simulink model "AdaptiveControlTrajectoryTracking"  (R2020b)
settings: Solver=VariableStepAuto  StartTime=0.0  StopTime=160  RelTol=1e-3
libraries: mobileRoboticsLib x4, simulink x4, dspinverses x4, dsppolyfun x4
settings Model: Creator=user  LastModifiedBy=user

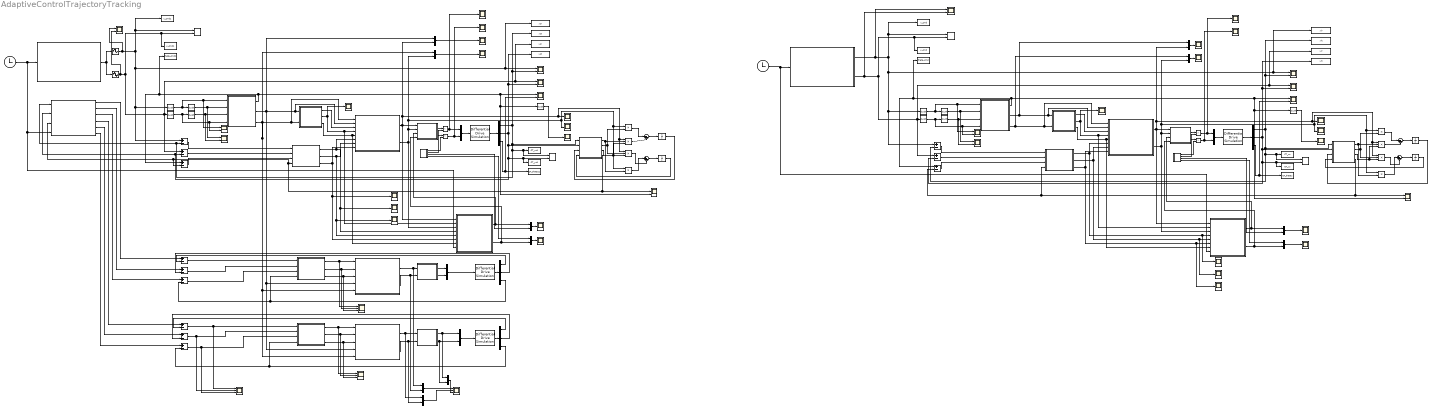
== system AdaptiveControlTrajectoryTracking ==
  Clock : Clock
  Clock1 : Clock
  Control law : MATLAB Function  TreatAsAtomicUnit=on
  Control law1 : MATLAB Function  TreatAsAtomicUnit=on
  Control law2 : MATLAB Function  TreatAsAtomicUnit=on
  Control law3 : MATLAB Function  TreatAsAtomicUnit=on
  Demux{1..4} (4 alike) : Demux  Outputs=3
  Derivative{1..10} (10 alike) : Derivative  CoefficientInTFapproximation=0
  Desired trajectory1 : MATLAB Function  TreatAsAtomicUnit=on
  Desired trajectory2 : MATLAB Function  TreatAsAtomicUnit=on
  Differential Drive Simulation1 : mobileRoboticsLib/Kinematic Models/Differential Drive/Differential Drive Simulation  wheelRadius=0.075  wheelBase=0.3  initX=0.05  initY=0.02  initAngle=pi-0.2  Ts=-1
      settings: SourceProductName=Mobile Robotics Simulation Toolbox
  Differential Drive Simulation2 : mobileRoboticsLib/Kinematic Models/Differential Drive/Differential Drive Simulation  wheelRadius=0.075  wheelBase=0.3  initX=0.2  initY=0.1  initAngle=pi  Ts=0.01
      settings: SourceProductName=Mobile Robotics Simulation Toolbox
  Differential Drive Simulation3 : mobileRoboticsLib/Kinematic Models/Differential Drive/Differential Drive Simulation  wheelRadius=0.075  wheelBase=0.3  initX=0.6  initY=-0.4  initAngle=pi  Ts=0.01
      settings: SourceProductName=Mobile Robotics Simulation Toolbox
  Differential Drive Simulation4 : mobileRoboticsLib/Kinematic Models/Differential Drive/Differential Drive Simulation  wheelRadius=0.075  wheelBase=0.3  initX=-0.15  initY=-0.13  initAngle=0  Ts=-1
      settings: SourceProductName=Mobile Robotics Simulation Toolbox
  Error1 : MATLAB Function  TreatAsAtomicUnit=on
  Error2 : MATLAB Function  TreatAsAtomicUnit=on
  Error3 : MATLAB Function  TreatAsAtomicUnit=on
  Error5 : MATLAB Function  TreatAsAtomicUnit=on
  Feedback gain1 : MATLAB Function  TreatAsAtomicUnit=on
  Feedback gain2 : MATLAB Function  TreatAsAtomicUnit=on
  Formation Control : MATLAB Function  TreatAsAtomicUnit=on
  Integrator : Integrator  InitialCondition=-100
  Integrator1 : Integrator  InitialCondition=1
  Integrator2 : Integrator  InitialCondition=800
  Integrator3 : Integrator  InitialCondition=200
  MATLAB Function1 : MATLAB Function  TreatAsAtomicUnit=on
  MATLAB Function2 : MATLAB Function  TreatAsAtomicUnit=on
  MATLAB Function3 : MATLAB Function  TreatAsAtomicUnit=on
  MATLAB Function4 : MATLAB Function  TreatAsAtomicUnit=on
  Mux{,1..11,14,17..18} (15 alike) : Mux  Inputs=2
  Observer : MATLAB Function  TreatAsAtomicUnit=on
  Observer slip{2..5} (4 alike) : Scope
  Observer theta : Scope  NumInputPorts=2
  Observer theta1 : Scope  NumInputPorts=2
  Observer theta3 : Scope
  Observer theta4 : Scope
  Observer1 : MATLAB Function  TreatAsAtomicUnit=on
  Product{,1..3,6..9} (8 alike) : Product
  Product{4..5,10..11} (4 alike) : Product  Inputs=3
  Scope{1,4,9..10} (4 alike) : Scope  NumInputPorts=2
  Scope{2..3,5..8,11..14} (10 alike) : Scope
  Subsystem1 : Subsystem
  Subsystem2 : Subsystem
  Subsystem3 : Subsystem
  Subsystem4 : Subsystem
  Sum : Sum  Inputs=|--
  Sum1 : Sum  Inputs=|+-
  Sum2 : Sum  Inputs=|--
  Sum3 : Sum  Inputs=|+-
  To Workspace : ToWorkspace  VariableName=xlr  SampleTime=.01
      settings: Save2DSignal=2-D array (concatenate along first dimension)
  To Workspace1 : ToWorkspace  VariableName=y_cmd  SampleTime=-1
      settings: Save2DSignal=2-D array (concatenate along first dimension)
  To Workspace10 : ToWorkspace  VariableName=y_cmd1  SampleTime=-1
      settings: Save2DSignal=2-D array (concatenate along first dimension)
  To Workspace11 : ToWorkspace  VariableName=theta_cmd1  SampleTime=-1
      settings: Save2DSignal=2-D array (concatenate along first dimension)
  To Workspace12 : ToWorkspace  VariableName=CT_thetas1  SampleTime=-1
      settings: Save2DSignal=2-D array (concatenate along first dimension)
  To Workspace13 : ToWorkspace  VariableName=xlt  SampleTime=.01
      settings: Save2DSignal=2-D array (concatenate along first dimension)
  To Workspace14 : ToWorkspace  VariableName=ylr  SampleTime=.01
      settings: Save2DSignal=2-D array (concatenate along first dimension)
  To Workspace15 : ToWorkspace  VariableName=ylt  SampleTime=.01
      settings: Save2DSignal=2-D array (concatenate along first dimension)
  To Workspace16 : ToWorkspace  VariableName=xcr  SampleTime=.01
      settings: Save2DSignal=2-D array (concatenate along first dimension)
  To Workspace17 : ToWorkspace  VariableName=xct  SampleTime=.01
      settings: Save2DSignal=2-D array (concatenate along first dimension)
  To Workspace18 : ToWorkspace  VariableName=ycr  SampleTime=.01
      settings: Save2DSignal=2-D array (concatenate along first dimension)
  To Workspace19 : ToWorkspace  VariableName=yct  SampleTime=.01
      settings: Save2DSignal=2-D array (concatenate along first dimension)
  To Workspace2 : ToWorkspace  VariableName=theta_cmd  SampleTime=-1
      settings: Save2DSignal=2-D array (concatenate along first dimension)
  To Workspace3 : ToWorkspace  VariableName=CT_xs1  SampleTime=-1
      settings: Save2DSignal=2-D array (concatenate along first dimension)
  To Workspace4 : ToWorkspace  VariableName=CT_ys1  SampleTime=-1
      settings: Save2DSignal=2-D array (concatenate along first dimension)
  To Workspace5 : ToWorkspace  VariableName=x_cmd1  SampleTime=-1
      settings: Save2DSignal=2-D array (concatenate along first dimension)
  To Workspace6 : ToWorkspace  VariableName=CT_thetas  SampleTime=-1
      settings: Save2DSignal=2-D array (concatenate along first dimension)
  To Workspace7 : ToWorkspace  VariableName=CT_xs  SampleTime=-1
      settings: Save2DSignal=2-D array (concatenate along first dimension)
  To Workspace8 : ToWorkspace  VariableName=CT_ys  SampleTime=-1
      settings: Save2DSignal=2-D array (concatenate along first dimension)
  To Workspace9 : ToWorkspace  VariableName=x_cmd  SampleTime=-1
      settings: Save2DSignal=2-D array (concatenate along first dimension)
  XY Graph desire1 : simulink/Sinks/XY Graph  xmin=-4  xmax=4  ymin=-4  ymax=4  st=-1
  XY Graph desire2 : simulink/Sinks/XY Graph  xmin=-1  xmax=10  ymin=-1  ymax=10  st=-1
  XY Graph tracking1 : simulink/Sinks/XY Graph  xmin=-4  xmax=4  ymin=-4  ymax=4  st=-1
  XY Graph tracking2 : simulink/Sinks/XY Graph  xmin=-1  xmax=10  ymin=-1  ymax=10  st=-1
  Xd1 : Sin  TimeSource=Use external signal  Amplitude=-1.6  SampleTime=0
  Yd1 : Sin  TimeSource=Use external signal  Amplitude=-1.6  Bias=1.6  Phase=pi/2  SampleTime=0
  angular velocity1 : Scope
  angular velocity2 : Scope
  dtheta1 : Scope
  dtheta2 : Scope
  e{1..4} (4 alike) : Scope
  error{1..4} (4 alike) : Scope  NumInputPorts=3
  left d1 : Scope  NumInputPorts=2
  left d2 : Scope  NumInputPorts=2
  theta1 : Scope  NumInputPorts=2
  theta2 : Scope  NumInputPorts=2
  theta_err{1..3,5} (4 alike) : Sum  Inputs=+-
  trajectory1 : Subsystem
  trajectory2 : Subsystem
  velocity1 : Scope
  velocity2 : Scope
  x1 : Scope  NumInputPorts=2
  x2 : Scope  NumInputPorts=2
  x_err{1..3,5} (4 alike) : Sum  Inputs=+-
  y1 : Scope  NumInputPorts=2
  y2 : Scope  NumInputPorts=2
  y_err{1..3,5} (4 alike) : Sum  Inputs=+-
  wires:
  Mux14/1 -> Observer slip2/1
  Mux/1 -> Observer slip3/1
  Subsystem2/1(ir) -> Product/2
  Feedback gain2/1(k1) -> Control law/3(k1)
  Mux1/1 -> Differential Drive Simulation1/1
  y_err2/1 -> Error2/2(y_err)
  Yd1/1 -> Scope10/2, To Workspace18/1, y2/1, Derivative5/1, y_err2/1, XY Graph desire1/2, To Workspace10/1
  Derivative5/1 -> Desired trajectory2/4(yd_d), left d1/2, Derivative8/1  "yd_d"
  Xd1/1 -> Scope10/1, To Workspace16/1, x2/1, Derivative4/1, x_err2/1, To Workspace5/1, XY Graph desire1/1
  Product/1 -> Mux1/2, Scope11/1
  Clock/1 -> Subsystem3/8(t), Formation Control/4(time), trajectory1/1(In1)
  Subsystem2/3(pl) -> Mux/2
  Subsystem3/1(Pl_hat) -> MATLAB Function1/3(Pl_hat), Mux/1
  theta_err2/1 -> Error2/3(theta_error)
  Desired trajectory2/1(td) -> To Workspace11/1, theta_err2/1, theta2/1, Observer theta/2, Derivative9/1
  Subsystem2/4(pr) -> Mux14/1
  Desired trajectory2/2(vd) -> Control law2/4(vd), Control law1/4(vd), Mux6/1, Feedback gain2/1(vd), Control law/2(vd)  "vr"
  Control law/1(v) -> MATLAB Function1/1(v), Product5/1, Product4/1, velocity1/1, Mux6/2, Subsystem3/1(v)  "v"
  Feedback gain2/2(k2) -> Scope14/1, Subsystem3/2(k2), Control law/4(k2)
  Product1/1 -> Mux1/1, Scope7/1
  MATLAB Function1/2(wr) -> Product/1  "wr"
  MATLAB Function1/1(wl) -> Product1/1  "wl"
  Differential Drive Simulation1/1 -> Demux1/1
  Subsystem2/2(il) -> Product1/2
  Derivative4/1 -> Derivative6/1, left d1/1, Desired trajectory2/1(xd_d)  "xd_d"
  Feedback gain2/3(k3) -> Control law/5(k3), Subsystem3/7(k3)
  Subsystem3/2(Pr_hat) -> MATLAB Function1/4(Pr_hat), Mux14/2
  trajectory1/1(Out1) -> Yd1/1, Xd1/1
  Derivative8/1 -> Scope9/2, Desired trajectory2/3(yd_dd)  "yd_dd"
  x_err2/1 -> Error2/1(x_err)
  Derivative6/1 -> Scope9/1, Desired trajectory2/2(xd_dd)  "xd_dd"
  Derivative9/1 -> dtheta1/1
  Control law/2(w) -> Mux7/2, Product3/1, Product2/1, angular velocity1/1, MATLAB Function1/2(w), Subsystem3/3(w)  "w"
  MATLAB Function2/1(wl) -> Mux2/1  "wl"
  MATLAB Function2/2(wr) -> Mux2/2  "wr"
  Control law1/1(v) -> MATLAB Function2/1(v), Mux4/1  "v"
  Control law1/2(w) -> MATLAB Function2/2(w), Mux4/2  "w"
  Differential Drive Simulation2/1 -> Demux2/1
  Control law2/2(w) -> Mux5/2, MATLAB Function3/2(w)  "w"
  Differential Drive Simulation3/1 -> Demux3/1
  Control law2/1(v) -> Mux5/1, MATLAB Function3/1(v)  "v"
  Error1/1(e1) -> error4/1, Control law1/1(ex)
  Error1/2(e2) -> error4/2, Control law1/2(ey)
  Error3/1(e1) -> error1/1, Control law2/1(ex)
  Error3/2(e2) -> error1/2, Control law2/2(ey)
  Error3/3(e3) -> error1/3, Control law2/3(et)
  x_err1/1 -> Error1/1(x_err)
  y_err1/1 -> Error1/2(y_err)
  theta_err1/1 -> Error1/3(theta_error)
  x_err3/1 -> error3/1, Error3/1(x_err)
  y_err3/1 -> error3/2, Error3/2(y_err)
  theta_err3/1 -> error3/3, Error3/3(theta_error)
  Demux3/3 -> Error3/4(theta), theta_err3/2
  Demux2/1 -> x_err1/2
  Demux2/2 -> y_err1/2
  Demux2/3 -> Error1/4(theta), theta_err1/2
  Formation Control/1(fx1) -> x_err1/1
  Formation Control/2(fy1) -> y_err1/1
  Formation Control/3(ft1) -> theta_err1/1
  Formation Control/4(fx2) -> x_err3/1
  Formation Control/5(fy2) -> y_err3/1
  Formation Control/6(fz2) -> theta_err3/1
  Mux4/1 -> error2/1
  Mux5/1 -> error2/2
  Demux1/1 -> XY Graph tracking1/1, To Workspace3/1, x_err2/2, Formation Control/1(Lx), Observer/1(z1), To Workspace17/1, x2/2
  Demux1/3 -> theta2/2, To Workspace12/1
  Demux1/2 -> To Workspace4/1, XY Graph tracking1/2, y_err2/2, Formation Control/2(Ly), Observer/2(z2), To Workspace19/1, y2/2
  Mux3/1 -> Differential Drive Simulation3/1
  Mux2/1 -> Differential Drive Simulation2/1
  MATLAB Function3/1(wl) -> Mux3/1, Mux8/1
  MATLAB Function3/2(wr) -> Mux3/2, Mux8/2
  Mux8/1 -> error2/3
  Demux3/2 -> y_err3/2
  Demux3/1 -> x_err3/2
  Error1/3(e3) -> error4/3, Control law1/3(et)
  Desired trajectory2/3(wd) -> Control law/1(wd), Feedback gain2/2(wd), Control law2/5(wd), Control law1/5(wd), Mux7/1  "wr"
  Observer/1(z3_hat) -> Product2/2, Product4/2
  Observer/3(L) -> Product5/3, Product4/3
  Observer/2(z4_hat) -> Product5/2, Product3/2
  Product3/1 -> Sum/1
  Product4/1 -> Sum/2
  Product2/1 -> Sum1/1
  Product5/1 -> Sum1/2
  Sum/1 -> Integrator/1
  Sum1/1 -> Integrator1/1
  Integrator/1 -> Observer/3(alpha)
  Integrator1/1 -> Observer/4(beta)
  Observer/4(theta) -> theta_err2/2, Formation Control/3(Lt), Error2/4(theta), Observer theta/1
  Demux4/3 -> theta1/2, To Workspace6/1
  trajectory2/2(Out2) -> y1/1, To Workspace14/1, Derivative2/1, y_err5/1, XY Graph desire2/2, To Workspace1/1, Scope1/2
  Demux4/1 -> XY Graph tracking2/1, To Workspace7/1, x_err5/2, Observer1/1(z1), x1/2, To Workspace13/1
  Demux4/2 -> To Workspace8/1, XY Graph tracking2/2, y_err5/2, Observer1/2(z2), y1/2, To Workspace15/1
  Mux10/1 -> Differential Drive Simulation4/1
  Subsystem4/2(Pr_hat) -> MATLAB Function4/4(Pr_hat), Mux11/2
  MATLAB Function4/1(wl) -> Product7/1  "wl"
  MATLAB Function4/2(wr) -> Product6/1  "wr"
  Derivative10/1 -> dtheta2/1
  Feedback gain1/2(k2) -> Scope2/1, Subsystem4/2(k2), Control law3/4(k2)
  trajectory2/1(Out1) -> Scope1/1, To Workspace9/1, XY Graph desire2/1, x1/1, To Workspace/1, Derivative1/1, x_err5/1
  Control law3/2(w) -> Mux18/2, Product9/1, Product8/1, angular velocity2/1, MATLAB Function4/2(w), Subsystem4/3(w)  "w"
  Desired trajectory1/1(td) -> To Workspace2/1, theta_err5/1, theta1/1, Observer theta1/2, Derivative10/1
  Error5/1(e1) -> e1/1, Subsystem4/4(e1), Control law3/6(e1)  "e1"
  x_err5/1 -> Error5/1(x_err)
  Subsystem4/1(Pl_hat) -> Mux9/1, MATLAB Function4/3(Pl_hat)
  Derivative7/1 -> Scope4/2, Desired trajectory1/3(yd_dd)  "yd_dd"
  Derivative3/1 -> Scope4/1, Desired trajectory1/2(xd_dd)  "xd_dd"
  Control law3/1(v) -> MATLAB Function4/1(v), Product11/1, Product10/1, velocity2/1, Mux17/2, Subsystem4/1(v)  "v"
  Differential Drive Simulation4/1 -> Demux4/1
  Subsystem1/4(pr) -> Mux11/1
  Feedback gain1/3(k3) -> Control law3/5(k3), Subsystem4/7(k3)
  Desired trajectory1/2(vd) -> Mux17/1, Feedback gain1/1(vd), Control law3/2(vd)  "vr"
  Derivative1/1 -> Derivative3/1, left d2/1, Desired trajectory1/1(xd_d)  "xd_d"
  Feedback gain1/1(k1) -> Control law3/3(k1)
  Error5/3(e3) -> Control law3/8(e3), Observer theta3/1, Subsystem4/6(e3)  "e3"
  Subsystem1/3(pl) -> Mux9/2
  Subsystem1/1(ir) -> Product6/2
  theta_err5/1 -> Error5/3(theta_error)
  Mux18/1 -> Scope5/1
  Observer1/4(theta) -> Error5/4(theta), theta_err5/2, Observer theta1/1
  Mux17/1 -> Scope3/1
  Integrator2/1 -> Observer1/3(alpha)
  Mux9/1 -> Observer slip5/1
  Derivative2/1 -> Desired trajectory1/4(yd_d), left d2/2, Derivative7/1  "yd_d"
  Subsystem1/2(il) -> Product7/2
  Clock1/1 -> Subsystem4/8(t), trajectory2/1(In1)
  Sum2/1 -> Integrator2/1
  Observer1/1(z3_hat) -> Product8/2, Product10/2
  Error5/2(e2) -> e2/1, Subsystem4/5(e2), Control law3/7(e2)  "e2"
  Sum3/1 -> Integrator3/1
  Mux11/1 -> Observer slip4/1
  Integrator3/1 -> Observer1/4(beta)
  Observer1/3(L) -> Product11/3, Product10/3
  Observer1/2(z4_hat) -> Product11/2, Product9/2
  Product8/1 -> Sum3/1
  Product11/1 -> Sum3/2
  y_err5/1 -> Error5/2(y_err)
  Product10/1 -> Sum2/2
  Product9/1 -> Sum2/1
  Desired trajectory1/3(wd) -> Control law3/1(wd), Feedback gain1/2(wd), Mux18/1  "wr"
  Error2/3(e3) -> Control law/8(e3), Subsystem3/6(e3), e3/1  "e3"
  Error2/1(e1) -> Subsystem3/4(e1), e4/1, Control law/6(e1)  "e1"
  Error2/2(e2) -> Control law/7(e2), Observer theta4/1, Subsystem3/5(e2)  "e2"
  Mux6/1 -> Scope6/1
  Mux7/1 -> Scope8/1
  Product6/1 -> Scope12/1, Mux10/2
  Product7/1 -> Scope13/1, Mux10/1

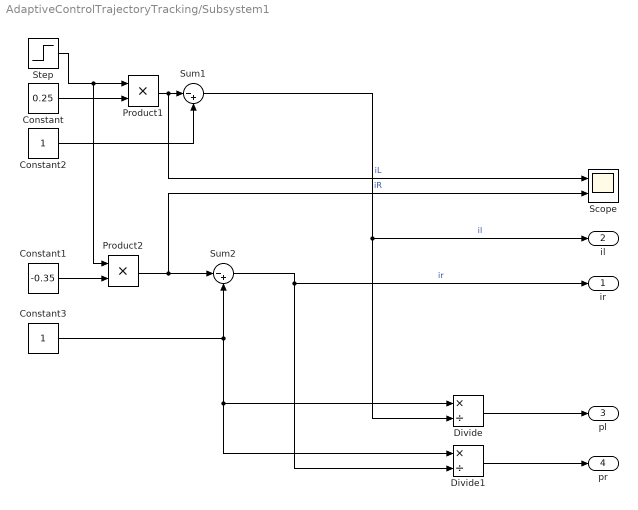
== system AdaptiveControlTrajectoryTracking/Subsystem1 ==
  Constant : Constant  Value=0.25
  Constant1 : Constant  Value=-0.35
  Constant2 : Constant
  Constant3 : Constant
  Divide : Product  Inputs=*/
  Divide1 : Product  Inputs=*/
  Product1 : Product
  Product2 : Product
  Scope : Scope  NumInputPorts=2
  Step : Step  Time=0  SampleTime=0
  Sum1 : Sum  Inputs=|-+
  Sum2 : Sum  Inputs=|-+
  ir : Outport
  il : Outport  Port=2
  pl : Outport  Port=3
  pr : Outport  Port=4
  wires:
  Sum1/1 -> Divide/2, il/1  "il"
  Step/1 -> Product2/1, Product1/1
  Constant3/1 -> Divide/1, Divide1/1, Sum2/2
  Product1/1 -> Scope/1, Sum1/1  "iL"
  Constant2/1 -> Sum1/2
  Sum2/1 -> ir/1, Divide1/2  "ir"
  Constant1/1 -> Product2/2
  Constant/1 -> Product1/2
  Product2/1 -> Scope/2, Sum2/1  "iR"
  Divide/1 -> pl/1
  Divide1/1 -> pr/1

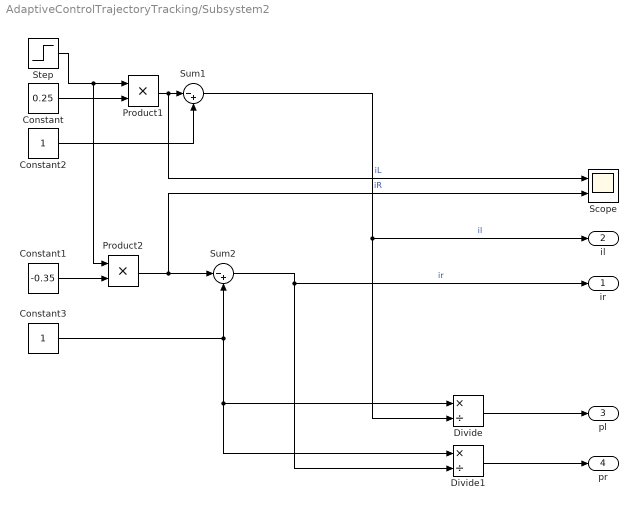
== system AdaptiveControlTrajectoryTracking/Subsystem2 ==
  Constant : Constant  Value=0.25
  Constant1 : Constant  Value=-0.35
  Constant2 : Constant
  Constant3 : Constant
  Divide : Product  Inputs=*/
  Divide1 : Product  Inputs=*/
  Product1 : Product
  Product2 : Product
  Scope : Scope  NumInputPorts=2
  Step : Step  Time=0  SampleTime=0
  Sum1 : Sum  Inputs=|-+
  Sum2 : Sum  Inputs=|-+
  ir : Outport
  il : Outport  Port=2
  pl : Outport  Port=3
  pr : Outport  Port=4
  wires:
  Sum1/1 -> Divide/2, il/1  "il"
  Step/1 -> Product2/1, Product1/1
  Constant3/1 -> Divide/1, Divide1/1, Sum2/2
  Product1/1 -> Scope/1, Sum1/1  "iL"
  Constant2/1 -> Sum1/2
  Sum2/1 -> ir/1, Divide1/2  "ir"
  Constant1/1 -> Product2/2
  Constant/1 -> Product1/2
  Product2/1 -> Scope/2, Sum2/1  "iR"
  Divide/1 -> pl/1
  Divide1/1 -> pr/1

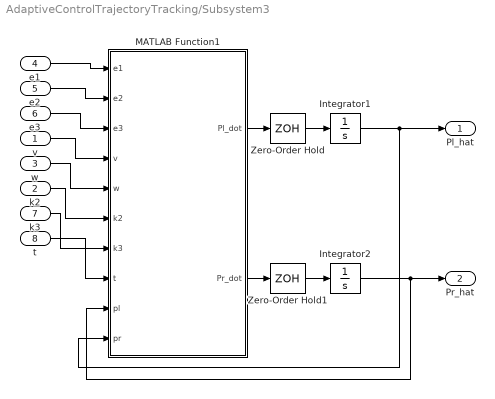
== system AdaptiveControlTrajectoryTracking/Subsystem3 ==
  v : Inport
  k2 : Inport  Port=2
  w : Inport  Port=3
  e1 : Inport  Port=4
  e2 : Inport  Port=5
  e3 : Inport  Port=6
  k3 : Inport  Port=7
  t : Inport  Port=8
  Integrator1 : Integrator  InitialCondition=1/0.85
  Integrator2 : Integrator  InitialCondition=1/1.2
  MATLAB Function1 : MATLAB Function  TreatAsAtomicUnit=on
  Zero-Order Hold : ZeroOrderHold  SampleTime=0.01
  Zero-Order Hold1 : ZeroOrderHold  SampleTime=0.01
  Pl_hat : Outport
  Pr_hat : Outport  Port=2
  wires:
  e2/1 -> MATLAB Function1/2(e2)
  Integrator1/1 -> Pl_hat/1, MATLAB Function1/10(pr)
  MATLAB Function1/2(Pr_dot) -> Zero-Order Hold1/1
  e3/1 -> MATLAB Function1/3(e3)
  w/1 -> MATLAB Function1/5(w)
  MATLAB Function1/1(Pl_dot) -> Zero-Order Hold/1
  k2/1 -> MATLAB Function1/6(k2)
  v/1 -> MATLAB Function1/4(v)
  e1/1 -> MATLAB Function1/1(e1)
  k3/1 -> MATLAB Function1/7(k3)
  Integrator2/1 -> Pr_hat/1, MATLAB Function1/9(pl)
  t/1 -> MATLAB Function1/8(t)
  Zero-Order Hold/1 -> Integrator1/1
  Zero-Order Hold1/1 -> Integrator2/1

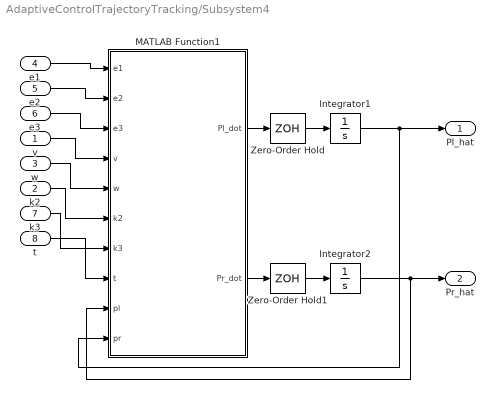
== system AdaptiveControlTrajectoryTracking/Subsystem4 ==
  v : Inport
  k2 : Inport  Port=2
  w : Inport  Port=3
  e1 : Inport  Port=4
  e2 : Inport  Port=5
  e3 : Inport  Port=6
  k3 : Inport  Port=7
  t : Inport  Port=8
  Integrator1 : Integrator  InitialCondition=1/0.85
  Integrator2 : Integrator  InitialCondition=1/1.2
  MATLAB Function1 : MATLAB Function  TreatAsAtomicUnit=on
  Zero-Order Hold : ZeroOrderHold  SampleTime=0.01
  Zero-Order Hold1 : ZeroOrderHold  SampleTime=0.01
  Pl_hat : Outport
  Pr_hat : Outport  Port=2
  wires:
  e2/1 -> MATLAB Function1/2(e2)
  Integrator1/1 -> Pl_hat/1, MATLAB Function1/10(pr)
  MATLAB Function1/2(Pr_dot) -> Zero-Order Hold1/1
  e3/1 -> MATLAB Function1/3(e3)
  w/1 -> MATLAB Function1/5(w)
  MATLAB Function1/1(Pl_dot) -> Zero-Order Hold/1
  k2/1 -> MATLAB Function1/6(k2)
  v/1 -> MATLAB Function1/4(v)
  e1/1 -> MATLAB Function1/1(e1)
  k3/1 -> MATLAB Function1/7(k3)
  Integrator2/1 -> Pr_hat/1, MATLAB Function1/9(pl)
  t/1 -> MATLAB Function1/8(t)
  Zero-Order Hold/1 -> Integrator1/1
  Zero-Order Hold1/1 -> Integrator2/1

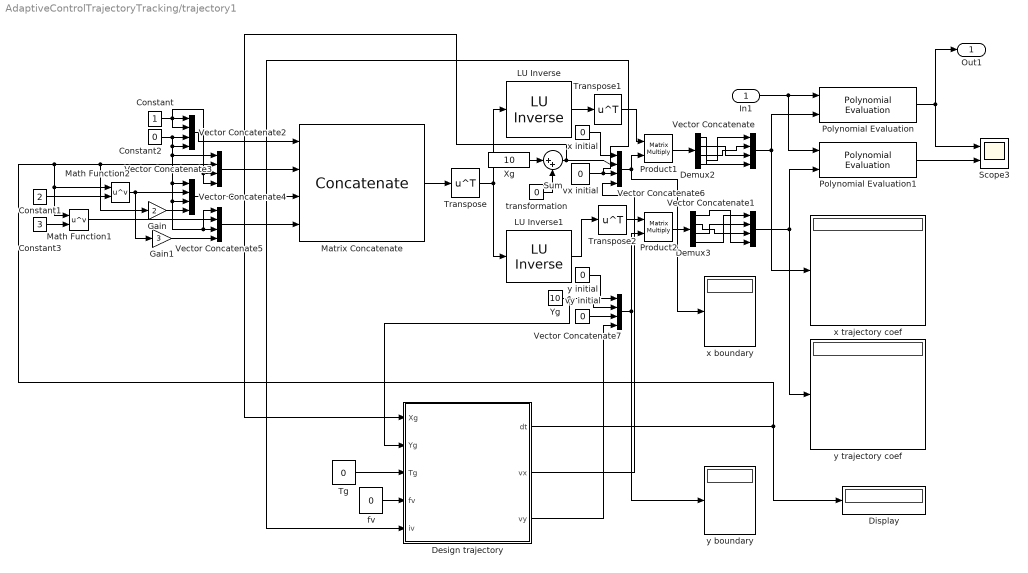
== system AdaptiveControlTrajectoryTracking/trajectory1 ==
  In1 : Inport
  " LU Inverse" : dspinverses/ LU Inverse
  " LU Inverse1" : dspinverses/ LU Inverse
  Constant : Constant
  Constant1 : Constant  Value=2
  Constant2 : Constant  Value=0
  Constant3 : Constant  Value=3
  Demux2 : Demux
  Demux3 : Demux
  Design trajectory : MATLAB Function  TreatAsAtomicUnit=on
  Display : Display
  Gain : Gain  Gain=2
  Gain1 : Gain  Gain=3
  Math Function1 : Math  Operator=pow  SaturateOnIntegerOverflow=on
  Math Function2 : Math  Operator=pow  SaturateOnIntegerOverflow=on
  Matrix Concatenate : Concatenate  NumInputs=4  Mode=Multidimensional array  ConcatenateDimension=2
  Polynomial Evaluation : dsppolyfun/Polynomial Evaluation  useConstCoeffs=off  constCoeffs=[5 4 3 2]
      settings: SourceProductBaseCode=DS
  Polynomial Evaluation1 : dsppolyfun/Polynomial Evaluation  useConstCoeffs=off  constCoeffs=[5 4 3 2]
      settings: SourceProductBaseCode=DS
  Product1 : Product  Multiplication=Matrix(*)
  Product2 : Product  Multiplication=Matrix(*)
  Scope3 : Scope  NumInputPorts=2
  Sum : Sum  Inputs=|++
  Tg : Constant  Value=0
  Transpose : Math  Operator=transpose  SaturateOnIntegerOverflow=on
  Transpose1 : Math  Operator=transpose  SaturateOnIntegerOverflow=on
  Transpose2 : Math  Operator=transpose  SaturateOnIntegerOverflow=on
  Vector Concatenate{,1..7} (8 alike) : Concatenate  NumInputs=4
  "Xg " : Constant  Value=10
  Yg : Constant  Value=10
  fv : Constant  Value=0
  transformation : Constant  Value=0
  "vx initial " : Constant  Value=0
  "vy initial " : Constant  Value=0
  "x boundary " : Display
  "x initial " : Constant  Value=0
  x trajectory coef : Display
  "y boundary " : Display
  "y initial " : Constant  Value=0
  y trajectory coef : Display
  Out1 : Outport
  wires:
  Polynomial Evaluation1/1 -> Scope3/2
  Product2/1 -> Demux3/1
  Yg/1 -> Design trajectory/2(Yg), Vector Concatenate7/2
  Math Function2/1 -> Gain1/1, Vector Concatenate4/2
  "vy initial "/1 -> Vector Concatenate7/3
  Tg/1 -> Design trajectory/3(Tg)
  Demux2/2 -> Vector Concatenate/3
  Constant/1 -> Vector Concatenate2/1, Vector Concatenate3/4, Vector Concatenate3/3, Vector Concatenate2/2
  fv/1 -> Design trajectory/4(fv)
  Vector Concatenate3/1 -> Matrix Concatenate/2
  Vector Concatenate5/1 -> Matrix Concatenate/4
  Vector Concatenate6/1 -> "x boundary "/1, Product1/2
  Vector Concatenate7/1 -> Product2/2, "y boundary "/1
  transformation/1 -> Sum/2
  Constant2/1 -> Vector Concatenate5/3, Vector Concatenate5/1, Vector Concatenate4/3, Vector Concatenate4/1, Vector Concatenate3/1, Vector Concatenate2/4, Vector Concatenate2/3
  Design trajectory/3(vy) -> Vector Concatenate7/4
  Transpose1/1 -> Product1/1
  "x initial "/1 -> Vector Concatenate6/1
  Demux3/4 -> Vector Concatenate1/1
  "Xg "/1 -> Sum/1
  " LU Inverse"/1 -> Transpose1/1
  " LU Inverse1"/1 -> Transpose2/1
  Product1/1 -> Demux2/1
  Vector Concatenate2/1 -> Matrix Concatenate/1
  "y initial "/1 -> Vector Concatenate7/1
  Demux2/3 -> Vector Concatenate/2
  Constant1/1 -> Math Function2/2
  Transpose2/1 -> Product2/1
  Matrix Concatenate/1 -> Transpose/1
  Vector Concatenate4/1 -> Matrix Concatenate/3
  Design trajectory/2(vx) -> Vector Concatenate6/4
  "vx initial "/1 -> Design trajectory/5(iv), Vector Concatenate6/3
  Polynomial Evaluation/1 -> Out1/1, Scope3/1
  Design trajectory/1(dt) -> Display/1, Math Function1/1, Math Function2/1, Vector Concatenate3/2, Gain/1
  Sum/1 -> Vector Concatenate6/2, Design trajectory/1(Xg)
  Transpose/1 -> " LU Inverse1"/1, " LU Inverse"/1
  In1/1 -> Polynomial Evaluation1/1, Polynomial Evaluation/1
  Constant3/1 -> Math Function1/2
  Math Function1/1 -> Vector Concatenate5/2
  Vector Concatenate1/1 -> y trajectory coef/1, Polynomial Evaluation1/2
  Gain/1 -> Vector Concatenate4/4
  Gain1/1 -> Vector Concatenate5/4
  Demux3/2 -> Vector Concatenate1/3
  Demux3/1 -> Vector Concatenate1/4
  Demux2/1 -> Vector Concatenate/4
  Demux3/3 -> Vector Concatenate1/2
  Vector Concatenate/1 -> x trajectory coef/1, Polynomial Evaluation/2
  Demux2/4 -> Vector Concatenate/1

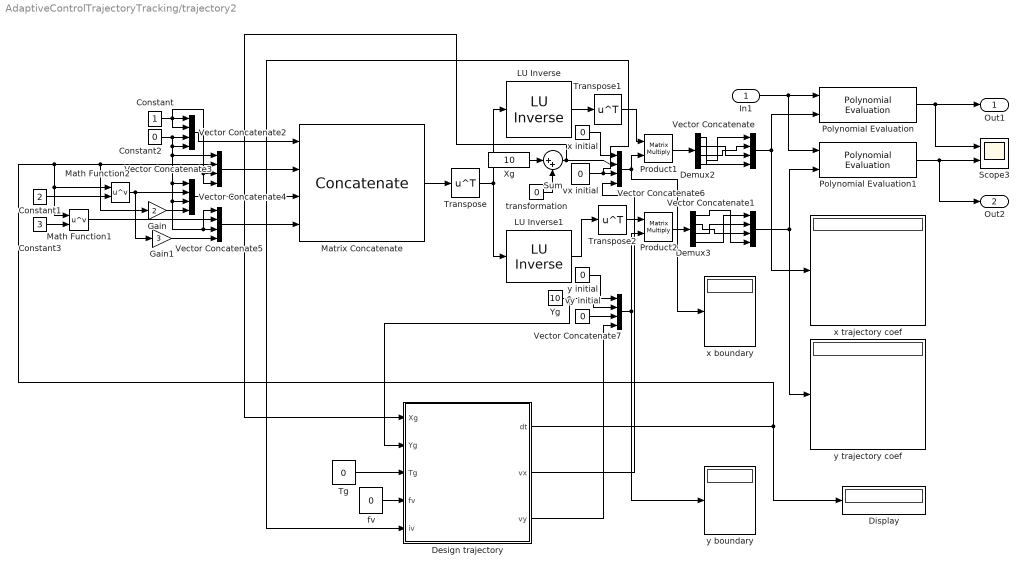
== system AdaptiveControlTrajectoryTracking/trajectory2 ==
  In1 : Inport
  " LU Inverse" : dspinverses/ LU Inverse
  " LU Inverse1" : dspinverses/ LU Inverse
  Constant : Constant
  Constant1 : Constant  Value=2
  Constant2 : Constant  Value=0
  Constant3 : Constant  Value=3
  Demux2 : Demux
  Demux3 : Demux
  Design trajectory : MATLAB Function  TreatAsAtomicUnit=on
  Display : Display
  Gain : Gain  Gain=2
  Gain1 : Gain  Gain=3
  Math Function1 : Math  Operator=pow  SaturateOnIntegerOverflow=on
  Math Function2 : Math  Operator=pow  SaturateOnIntegerOverflow=on
  Matrix Concatenate : Concatenate  NumInputs=4  Mode=Multidimensional array  ConcatenateDimension=2
  Polynomial Evaluation : dsppolyfun/Polynomial Evaluation  useConstCoeffs=off  constCoeffs=[5 4 3 2]
      settings: SourceProductBaseCode=DS
  Polynomial Evaluation1 : dsppolyfun/Polynomial Evaluation  useConstCoeffs=off  constCoeffs=[5 4 3 2]
      settings: SourceProductBaseCode=DS
  Product1 : Product  Multiplication=Matrix(*)
  Product2 : Product  Multiplication=Matrix(*)
  Scope3 : Scope  NumInputPorts=2
  Sum : Sum  Inputs=|++
  Tg : Constant  Value=0
  Transpose : Math  Operator=transpose  SaturateOnIntegerOverflow=on
  Transpose1 : Math  Operator=transpose  SaturateOnIntegerOverflow=on
  Transpose2 : Math  Operator=transpose  SaturateOnIntegerOverflow=on
  Vector Concatenate{,1..7} (8 alike) : Concatenate  NumInputs=4
  "Xg " : Constant  Value=10
  Yg : Constant  Value=10
  fv : Constant  Value=0
  transformation : Constant  Value=0
  "vx initial " : Constant  Value=0
  "vy initial " : Constant  Value=0
  "x boundary " : Display
  "x initial " : Constant  Value=0
  x trajectory coef : Display
  "y boundary " : Display
  "y initial " : Constant  Value=0
  y trajectory coef : Display
  Out1 : Outport
  Out2 : Outport  Port=2
  wires:
  Polynomial Evaluation1/1 -> Scope3/2, Out2/1
  Product2/1 -> Demux3/1
  Yg/1 -> Design trajectory/2(Yg), Vector Concatenate7/2
  Math Function2/1 -> Gain1/1, Vector Concatenate4/2
  "vy initial "/1 -> Vector Concatenate7/3
  Tg/1 -> Design trajectory/3(Tg)
  Demux2/2 -> Vector Concatenate/3
  Constant/1 -> Vector Concatenate2/1, Vector Concatenate3/4, Vector Concatenate3/3, Vector Concatenate2/2
  fv/1 -> Design trajectory/4(fv)
  Vector Concatenate3/1 -> Matrix Concatenate/2
  Vector Concatenate5/1 -> Matrix Concatenate/4
  Vector Concatenate6/1 -> "x boundary "/1, Product1/2
  Vector Concatenate7/1 -> Product2/2, "y boundary "/1
  transformation/1 -> Sum/2
  Constant2/1 -> Vector Concatenate5/3, Vector Concatenate5/1, Vector Concatenate4/3, Vector Concatenate4/1, Vector Concatenate3/1, Vector Concatenate2/4, Vector Concatenate2/3
  Design trajectory/3(vy) -> Vector Concatenate7/4
  Transpose1/1 -> Product1/1
  "x initial "/1 -> Vector Concatenate6/1
  Demux3/4 -> Vector Concatenate1/1
  "Xg "/1 -> Sum/1
  " LU Inverse"/1 -> Transpose1/1
  " LU Inverse1"/1 -> Transpose2/1
  Product1/1 -> Demux2/1
  Vector Concatenate2/1 -> Matrix Concatenate/1
  "y initial "/1 -> Vector Concatenate7/1
  Demux2/3 -> Vector Concatenate/2
  Constant1/1 -> Math Function2/2
  Transpose2/1 -> Product2/1
  Matrix Concatenate/1 -> Transpose/1
  Vector Concatenate4/1 -> Matrix Concatenate/3
  Design trajectory/2(vx) -> Vector Concatenate6/4
  "vx initial "/1 -> Design trajectory/5(iv), Vector Concatenate6/3
  Polynomial Evaluation/1 -> Out1/1, Scope3/1
  Design trajectory/1(dt) -> Display/1, Math Function1/1, Math Function2/1, Vector Concatenate3/2, Gain/1
  Sum/1 -> Vector Concatenate6/2, Design trajectory/1(Xg)
  Transpose/1 -> " LU Inverse1"/1, " LU Inverse"/1
  In1/1 -> Polynomial Evaluation1/1, Polynomial Evaluation/1
  Constant3/1 -> Math Function1/2
  Math Function1/1 -> Vector Concatenate5/2
  Vector Concatenate1/1 -> y trajectory coef/1, Polynomial Evaluation1/2
  Gain/1 -> Vector Concatenate4/4
  Gain1/1 -> Vector Concatenate5/4
  Demux3/2 -> Vector Concatenate1/3
  Demux3/1 -> Vector Concatenate1/4
  Demux2/1 -> Vector Concatenate/4
  Demux3/3 -> Vector Concatenate1/2
  Vector Concatenate/1 -> x trajectory coef/1, Polynomial Evaluation/2
  Demux2/4 -> Vector Concatenate/1

== matlab function AdaptiveControlTrajectoryTracking/Error3 ==
  data: x_err input; e1 output; y_err input; theta_error input; theta input; e2 output; e3 output
function [e1,e2,e3] = error(x_err,y_err,theta_error,theta)
    e=[cos(theta) sin(theta) 0;-sin(theta) cos(theta) 0;0 0 1]*[x_err;y_err;theta_error];
    e1=e(1);
    e2=e(2);
    e3=e(3);
end

== matlab function AdaptiveControlTrajectoryTracking/Error2 ==
  data: x_err input; e1 output; y_err input; theta_error input; theta input; e2 output; e3 output
function [e1,e2,e3] = error(x_err,y_err,theta_error,theta)
    e=[cos(theta) sin(theta) 0;-sin(theta) cos(theta) 0;0 0 1]*[x_err;y_err;theta_error];
    e1=e(1);
    e2=e(2);
    e3=e(3);
end

== matlab function AdaptiveControlTrajectoryTracking/Feedback gain2 ==
  data: k1 output; k2 output; k3 output; vd input; wd input
function [k1,k2,k3] = K(vd,wd)
    epsilon=1;
    kb=14;
    
    k1=2*epsilon*sqrt(wd^2+kb*vd^2);
    k3=k1;
    k2=kb*abs(vd);

end

== matlab function AdaptiveControlTrajectoryTracking/Control law ==
  data: wd input; vd input; v output; k1 input; k2 input; k3 input; e1 input; e2 input; e3 input; w output
function [v,w] = fcn(wd,vd,k1,k2,k3,e1,e2,e3)
    v=zeros(1);
    w=zeros(1);
    vmax=0.15;
    wmax=0.45;
    
    
%    vc=vd*cos(e3)+k1*e1;
%    wc=wd+k2*sign(vd)*e2+k3*e3;
    
    %% gain 
    
    k11 = 2;
    k22 = 10;
    k33 = 2;
    
    %%
    wc = wd + vd / 2 * (k22 * (e2 + k33 * e3) + sin(e3) / k33); 
    vc = vd * cos(e3) + k33 * e3 * wc + k11 * e1;
%     wc=wd+k2*(vd)*e2+k3*sin(e3);

    sigma=max([abs(vc/vmax),abs(wc/wmax),1]);
    if(sigma==1)
        v=vc;
        w=wc;
    elseif(sigma==vc/vmax)
        v=sign(vc)*vmax;
        w=wc/sigma;
    else
        v=vc/sigma;
        w=sign(wc)*wmax;

    end
end

== matlab function AdaptiveControlTrajectoryTracking/MATLAB Function1 ==
  data: v input; wl output; w input; Pl_hat input; Pr_hat input; wr output
function [wl,wr] = IK(v,w,Pl_hat,Pr_hat)
    %parameters
    r=0.075;
    b=0.3;
    %inverse kinematics
%     wl = v/(r*il) - w*b/(r*il);
%     wr = v/(r*ir) + w*b/(r*ir);
    wl = v*Pl_hat/(r) - w*b*Pl_hat/(2*r);
    wr = v*Pr_hat/(r) + w*b*Pr_hat/(2*r);
end

== matlab function AdaptiveControlTrajectoryTracking/Subsystem3/MATLAB Function1 ==
  data: e1 input; Pl_dot output; e2 input; e3 input; v input; w input; Pr_dot output; k2 input; k3 input; t input; pl input; pr input
function [Pl_dot,Pr_dot]  = observer(e1,e2,e3,v,w,k2,k3, t,pl, pr)
%% Paramaters
    gamma1 = 0.4;
    gamma2 = 0.4;
    r=0.075;
    b=0.3;
    k1 = 2;
    k2 = 10;
    k3 = 2;

        Pl_dot = gamma1 * (v - b*w/2) * (e1 * (e2/b + 1/2) - e1 * (e2 + k3 * e3)/b - k3 * (e2 + k3 * e3) / b - sin(e3)/(b*k2));
        Pr_dot = gamma2 * (v + b*w/2) * (-e1 * (e2/b - 1/2) + e1 * (e2 + k3 * e3)/b + k3 * (e2 + k3 * e3) / b + sin(e3)/(b*k2));
%%
%     %parameters
%     r=0.075;
%     b=0.3;
%     p1=5;
%     p2=5;
% 
%     if (t<0.1)
%         iLdot=1;
%         iRdot=1;
%     else
%         iLdot=p1*((e2/b + 1/2)*e1*v - (e2/2 + b/4)*e1*w - sin(e3)/k2*(v/b - w/2));
%         iRdot=p2*(-(e2/b - 1/2)*e1*v - (e2/2 - b/4)*e1*w + sin(e3)/k2*(v/b + w/2));
% 
%     end


end

== matlab function AdaptiveControlTrajectoryTracking/trajectory1/Design trajectory ==
  data: Xg input; dt output; Yg input; Tg input; fv input; vx output; vy output; iv input
function [dt,vx,vy] = cmd_generation(Xg,Yg,Tg,fv,iv)

    distance = sqrt(Xg*Xg + Yg*Yg);
%     distance = 1.6*Xg;
    vx = sqrt((fv*fv)/(1+tan(Tg)*tan(Tg)));
    vy = vx*tan(Tg);
    dt = distance/0.05;
end

== matlab function AdaptiveControlTrajectoryTracking/Control law3 ==
  data: wd input; vd input; v output; k1 input; k2 input; k3 input; e1 input; e2 input; e3 input; w output
function [v,w] = fcn(wd,vd,k1,k2,k3,e1,e2,e3)
    v=zeros(1);
    w=zeros(1);
    vmax=0.15;
    wmax=0.45;
    
    
%    vc=vd*cos(e3)+k1*e1;
%    wc=wd+k2*sign(vd)*e2+k3*e3;
    
    %% gain 
    
    k11 = 2;
    k22 = 10;
    k33 = 2;
    
    %%
    wc = wd + vd / 2 * (k22 * (e2 + k33 * e3) + sin(e3) / k33); 
    vc = vd * cos(e3) + k33 * e3 * wc + k11 * e1;
%     wc=wd+k2*(vd)*e2+k3*sin(e3);

    sigma=max([abs(vc/vmax),abs(wc/wmax),1]);
    if(sigma==1)
        v=vc;
        w=wc;
    elseif(sigma==vc/vmax)
        v=sign(vc)*vmax;
        w=wc/sigma;
    else
        v=vc/sigma;
        w=sign(wc)*wmax;

    end
end

== matlab function AdaptiveControlTrajectoryTracking/Desired trajectory1 ==
  data: xd_d input; td output; xd_dd input; yd_dd input; yd_d input; vd output; wd output
function [td,vd,wd] = cmd_generation(xd_d,xd_dd,yd_dd,yd_d)
%    if atan2(yd_d,xd_d)<0
%        td=atan2(yd_d,xd_d)+2*pi;
%    else
        td=atan2(yd_d,xd_d);
%    end
    vd = sqrt(xd_d^2+yd_d^2);
    if(xd_d^2+yd_d^2==0)
        wd=0;
    else
        wd=(yd_dd*xd_d-xd_dd*yd_d)/(xd_d^2+yd_d^2);
    end
end

== matlab function AdaptiveControlTrajectoryTracking/Error5 ==
  data: x_err input; e1 output; y_err input; theta_error input; theta input; e2 output; e3 output
function [e1,e2,e3] = error(x_err,y_err,theta_error,theta)
    e=[cos(theta) sin(theta) 0;-sin(theta) cos(theta) 0;0 0 1]*[x_err;y_err;theta_error];
    e1=e(1);
    e2=e(2);
    e3=e(3);
end

== matlab function AdaptiveControlTrajectoryTracking/Observer ==
  data: z3_hat output; z4_hat output; z1 input; z2 input; alpha input; beta input; L output; theta output
function [z3_hat,z4_hat,L,theta] = K(z1,z2,alpha,beta)
    L = 100;
    z3_hat = alpha + L * z1;
    z4_hat = beta + L * z2;
    theta = atan2(z4_hat,z3_hat);
end

== matlab function AdaptiveControlTrajectoryTracking/Feedback gain1 ==
  data: k1 output; k2 output; k3 output; vd input; wd input
function [k1,k2,k3] = K(vd,wd)
    epsilon=1;
    kb=14;
    
    k1=2*epsilon*sqrt(wd^2+kb*vd^2);
    k3=k1;
    k2=kb*abs(vd);

end

== matlab function AdaptiveControlTrajectoryTracking/MATLAB Function4 ==
  data: v input; wl output; w input; Pl_hat input; Pr_hat input; wr output
function [wl,wr] = IK(v,w,Pl_hat,Pr_hat)
    %parameters
    r=0.075;
    b=0.3;
    %inverse kinematics
%     wl = v/(r*il) - w*b/(r*il);
%     wr = v/(r*ir) + w*b/(r*ir);
    wl = v*Pl_hat/(r) - w*b*Pl_hat/(2*r);
    wr = v*Pr_hat/(r) + w*b*Pr_hat/(2*r);
end

== matlab function AdaptiveControlTrajectoryTracking/Control law1 ==
  data: ex input; ey input; v output; et input; vd input; wd input; w output
function [v,w] = fcn(ex,ey,et,vd,wd)
    q1 = 0.1;
    q2 = 0.1;
    q3 = 0.05;
    k3 = 0.1+q3;
    k2 = 0.1+vd*sin(et)/et;
    k1 = 0.1+q1+q2*ey*ey/(ex*ex);
%     ratio = 0.5;
%     vd = vd * ratio;
%     wd = wd * ratio;
    if(et == 0)
        v = vd * cos(et) + k1 * ex;
        w = wd + k3 * et + k2 * vd * ey;
    else
        v = vd * cos(et) + k1 * ex;
        w = wd + k3 * et + k2 * vd * ey * sin(et)/et;
    end

end

== matlab function AdaptiveControlTrajectoryTracking/Observer1 ==
  data: z3_hat output; z4_hat output; z1 input; z2 input; alpha input; beta input; L output; theta output
function [z3_hat,z4_hat,L,theta] = K(z1,z2,alpha,beta)
    L = 100;
    z3_hat = alpha + L * z1;
    z4_hat = beta + L * z2;
    theta = atan2(z4_hat,z3_hat);
end

== matlab function AdaptiveControlTrajectoryTracking/Subsystem4/MATLAB Function1 ==
  data: e1 input; Pl_dot output; e2 input; e3 input; v input; w input; Pr_dot output; k2 input; k3 input; t input; pl input; pr input
function [Pl_dot,Pr_dot]  = observer(e1,e2,e3,v,w,k2,k3, t,pl, pr)
%% Paramaters
    gamma1 = 0.05;
    gamma2 = 0.05;
    r=0.075;
    b=0.3;
    k1 = 2;
    k2 = 10;
    k3 = 2;

        Pl_dot = gamma1 * (v - b*w/2) * (e1 * (e2/b + 1/2) - e1 * (e2 + k3 * e3)/b - k3 * (e2 + k3 * e3) / b - sin(e3)/(b*k2));
        Pr_dot = gamma2 * (v + b*w/2) * (-e1 * (e2/b - 1/2) + e1 * (e2 + k3 * e3)/b + k3 * (e2 + k3 * e3) / b + sin(e3)/(b*k2));
%%
%     %parameters
%     r=0.075;
%     b=0.3;
%     p1=5;
%     p2=5;
% 
%     if (t<0.1)
%         iLdot=1;
%         iRdot=1;
%     else
%         iLdot=p1*((e2/b + 1/2)*e1*v - (e2/2 + b/4)*e1*w - sin(e3)/k2*(v/b - w/2));
%         iRdot=p2*(-(e2/b - 1/2)*e1*v - (e2/2 - b/4)*e1*w + sin(e3)/k2*(v/b + w/2));
% 
%     end


end

== matlab function AdaptiveControlTrajectoryTracking/trajectory2/Design trajectory ==
  data: Xg input; dt output; Yg input; Tg input; fv input; vx output; vy output; iv input
function [dt,vx,vy] = cmd_generation(Xg,Yg,Tg,fv,iv)

    distance = sqrt(Xg*Xg + Yg*Yg);
%     distance = 1.6*Xg;
    vx = sqrt((fv*fv)/(1+tan(Tg)*tan(Tg)));
    vy = vx*tan(Tg);
    dt = distance/0.05;
end

== matlab function AdaptiveControlTrajectoryTracking/MATLAB Function2 ==
  data: v input; wl output; w input; wr output
function [wl,wr] = IK(v,w)
    %parameters
    r=0.075;
    b=0.3;
    %inverse kinematics
%     wl = v/(r*il) - w*b/(r*il);
%     wr = v/(r*ir) + w*b/(r*ir);
    wl = v/(r) - w*b/(2*r);
    wr = v/(r) + w*b/(2*r);
end

== matlab function AdaptiveControlTrajectoryTracking/Formation Control ==
  data: Lx input; Ly input; fx1 output; Lt input; time input; fy1 output; ft1 output; fx2 output; fy2 output; fz2 output
function [fx1,fy1, ft1, fx2, fy2, fz2] = fcn(Lx,Ly,Lt,time)
    % Triangle Formation 
    if(time < 60)
        
        d = 0.3;
        theta1 = 3.14159/1.5;
        theta2 = 3.14159*3/2;
%         theta3 = ;
        %% First Robot
        fx1 = Lx + d * cos(Lt + theta1);
        fy1 = Ly + d * sin(Lt + theta1);
        ft1 = Lt;
        %% Second Roboe
        fx2 = Lx + d * cos(Lt + theta2);
        fy2 = Ly + d * sin(Lt + theta2);
        fz2 = Lt;
%         %% Third Robot
%         fx3 = Lx + d * cos(Lt + theta2);
%         fy3 = Ly + d * sin(Lt + theta2);
%         fz3 = Lt; 

    
    %Linear Formation
    elseif(time >= 60 && time < 120)
    
        d = 0.15;
        theta = 3.14159;
        
        fx1 = Lx + d * cos(Lt + theta);
        fy1 = Ly + d * sin(Lt + theta);
        ft1 = Lt;
        fx2 = Lx + d * 2 * cos(Lt + theta);
        fy2 = Ly + d * 2 * sin(Lt + theta);
        fz2 = ft1;
        
    
    % Closer Linear Formation
    else
    
        d = 0.1;
        theta = 3.14159;
              
        fx1 = Lx + d * cos(Lt + theta);
        fy1 = Ly + d * sin(Lt + theta);
        ft1 = Lt;
        fx2 = Lx + d * 2 * cos(Lt + theta);
        fy2 = Ly + d * 2 * sin(Lt + theta);
        fz2 = ft1;
    
        
    end


end

% function Linear_Geometry[] = fcn ()
%     G = graph([leader_x,leader_y],[])
% end
% function Triangular_Geometry[] = fcn() 
%     
% end
% 
% function SBOS[x,y,t] = fcn(l1,l2,beta,leader1_x,leader1_y,leader1_t,leader2_x,leader2_y,leader_t) % one connection, beta is the desire angular
% 
% end
% 
% function SSOS[x,y,t] = fcn(d,theta,leader_x,leader_y,leader_t) % two connection
%     x = leader_x + d * cos(leader_t + theta);
%     y = leader_y + d * sin(leader_t + theta);
%     t = theta;
% 
% end

== matlab function AdaptiveControlTrajectoryTracking/Desired trajectory2 ==
  data: xd_d input; td output; xd_dd input; yd_dd input; yd_d input; vd output; wd output
function [td,vd,wd] = cmd_generation(xd_d,xd_dd,yd_dd,yd_d)
%    if atan2(yd_d,xd_d)<0
%        td=atan2(yd_d,xd_d)+2*pi;
%    else
        td=atan2(yd_d,xd_d);
%    end
    vd = sqrt(xd_d^2+yd_d^2);
    if(xd_d^2+yd_d^2==0)
        wd=0;
    else
        wd=(yd_dd*xd_d-xd_dd*yd_d)/(xd_d^2+yd_d^2);
    end
end

== matlab function AdaptiveControlTrajectoryTracking/Control law2 ==
  data: ex input; ey input; v output; et input; vd input; wd input; w output
function [v,w] = fcn(ex,ey,et,vd,wd)
    q1 = 0.1;
    q2 = 0.1;
    q3 = 0.05;
    k3 = 0.1+q3;
    k2 = 0.1+vd*sin(et)/et;
    k1 = 0.1+q1+q2*ey*ey/(ex*ex);
%     ratio = 0.5;
%     vd = vd * ratio;
%     wd = wd * ratio;
    if(et == 0)
        v = vd * cos(et) + k1 * ex;
        w = wd + k3 * et + k2 * vd * ey;
    else
        v = vd * cos(et) + k1 * ex;
        w = wd + k3 * et + k2 * vd * ey * sin(et)/et;
    end

end

== matlab function AdaptiveControlTrajectoryTracking/Error1 ==
  data: x_err input; e1 output; y_err input; theta_error input; theta input; e2 output; e3 output
function [e1,e2,e3] = error(x_err,y_err,theta_error,theta)
    e=[cos(theta) sin(theta) 0;-sin(theta) cos(theta) 0;0 0 1]*[x_err;y_err;theta_error];
    e1=e(1);
    e2=e(2);
    e3=e(3);
end

== matlab function AdaptiveControlTrajectoryTracking/MATLAB Function3 ==
  data: v input; wl output; w input; wr output
function [wl,wr] = IK(v,w)
    %parameters
    r=0.075;
    b=0.3;
    %inverse kinematics
%     wl = 0.1;
%     wr = 0.1;
    wl = v/(r) - w*b/(2*r);
    wr = v/(r) + w*b/(2*r);
end
